simulink model "NLPIDVersion2"  (Simulink 7.3)
settings: Solver=ode5  StartTime=0.0  StopTime=inf  FixedStep=0.1  RelTol=1e-3
undefined symbols (not defined in the file): eta1_0_real, v1_0_real, velocitySatValues1
libraries: dspmtrx3 x16, simulink x14, dspindex x5, marine_gnc x4, simulink_extras x1, dspinverses x1
(part 4 of 4)

== system NLPIDVersion2/Main Subsystems/Guidance/Line-Of-Sight Path-Following/Path/Ellipse path/p_d^s^2 eq ==
  s : Inport
  r_x : Inport  Port=2
  r_y : Inport  Port=3
  k : Inport  Port=4
  Gain : Gain  Gain=-1  ParameterDataType=fixdt(1, 16)  ParameterScaling=2^0  OutDataType=fixdt(1, 16)  OutScaling=2^0
  Gain1 : Gain  Gain=-1  ParameterDataType=fixdt(1, 16)  ParameterScaling=2^0  OutDataType=fixdt(1, 16)  OutScaling=2^0
  Math Function : Math  Operator=square  OutDataType=fixdt(1, 16)  OutScaling=2^0  SaturateOnIntegerOverflow=on
  Mux2 : Mux  Inputs=2
  Product : Product  Inputs=3  OutDataType=fixdt(1, 16)  OutScaling=2^0  RndMeth=Zero
  Product1 : Product  Inputs=3  OutDataType=fixdt(1, 16)  OutScaling=2^0  RndMeth=Zero
  Product2 : Product  OutDataType=fixdt(1, 16)  OutScaling=2^0  RndMeth=Zero
  cos(s) : Trigonometry  Operator=cos
  sin(s) : Trigonometry
  p_d^s^2 : Outport
  wires:
  Math Function/1 -> Product/3, Product1/3
  Product2/1 -> sin(s)/1, cos(s)/1
  s/1 -> Product2/1
  k/1 -> Math Function/1, Product2/2
  r_x/1 -> Product/1
  r_y/1 -> Product1/1
  Mux2/1 -> p_d^s^2/1
  sin(s)/1 -> Product1/2
  cos(s)/1 -> Product/2
  Gain1/1 -> Mux2/2
  Product1/1 -> Gain1/1
  Gain/1 -> Mux2/1
  Product/1 -> Gain/1

== system NLPIDVersion2/Main Subsystems/Guidance/Line-Of-Sight Path-Following/Path/Ellipse path/p_d^s^3 eq ==
  s : Inport
  r_x : Inport  Port=2
  r_y : Inport  Port=3
  k : Inport  Port=4
  Constant : Constant  Value=3  OutDataType=fixdt(1, 16)  OutScaling=2^0
  Gain : Gain  Gain=-1  ParameterDataType=fixdt(1, 16)  ParameterScaling=2^0  OutDataType=fixdt(1, 16)  OutScaling=2^0
  Math Function : Math  Operator=pow  OutDataType=fixdt(1, 16)  OutScaling=2^0  SaturateOnIntegerOverflow=on
  Mux3 : Mux  Inputs=2
  Product : Product  Inputs=3  OutDataType=fixdt(1, 16)  OutScaling=2^0  RndMeth=Zero
  Product1 : Product  Inputs=3  OutDataType=fixdt(1, 16)  OutScaling=2^0  RndMeth=Zero
  Product2 : Product  OutDataType=fixdt(1, 16)  OutScaling=2^0  RndMeth=Zero
  cos(s)3 : Trigonometry  Operator=cos
  sin(s)3 : Trigonometry
  p_d^s^3 : Outport
  wires:
  Math Function/1 -> Product/3, Product1/3
  Constant/1 -> Math Function/2
  Product2/1 -> cos(s)3/1, sin(s)3/1
  s/1 -> Product2/1
  k/1 -> Math Function/1, Product2/2
  r_y/1 -> Product1/1
  r_x/1 -> Product/1
  sin(s)3/1 -> Product/2
  cos(s)3/1 -> Product1/2
  Product/1 -> Mux3/1
  Mux3/1 -> p_d^s^3/1
  Gain/1 -> Mux3/2
  Product1/1 -> Gain/1

== system NLPIDVersion2/Main Subsystems/Guidance/Line-Of-Sight Path-Following/Path/Ellipse path/|p_d^s| eq ==
  p_d^s : Inport
  Product : Product  Multiplication=Matrix(*)  OutDataType=fixdt(1, 16)  OutScaling=2^0  RndMeth=Zero
  p_d^s^T : dspmtrx3/Transpose  SystemSampleTime=-1  Hermitian=off  overflowFlag=off
  sqrt : Math  Operator=sqrt  OutDataType=fixdt(1, 16)  OutScaling=2^0  SaturateOnIntegerOverflow=on
  |p_d^s| : Outport
  wires:
  p_d^s^T/1 -> Product/1
  Product/1 -> sqrt/1
  sqrt/1 -> |p_d^s|/1
  p_d^s/1 -> p_d^s^T/1, Product/2

== system NLPIDVersion2/Main Subsystems/Guidance/Line-Of-Sight Path-Following/Path/Path Switch workaround + limiter/Limiter ==
  p_d : Inport  OutDataType=sfix(16)  OutScaling=2^0
  Demux : Demux  Outputs=2
  Mux1 : Mux  Inputs=2
  Saturation x : simulink/Discontinuities/Saturation Dynamic  SystemSampleTime=-1  OutMin=[]  OutMax=[]  OutDataTypeStr=Inherit: Same as second input  OutDataType=fixdt(1, 16)  OutScaling=2^-10  DoSatur=off
  Saturation y : simulink/Discontinuities/Saturation Dynamic  SystemSampleTime=-1  OutMin=[]  OutMax=[]  OutDataTypeStr=Inherit: Same as second input  OutDataType=fixdt(1, 16)  OutScaling=2^-10  DoSatur=off
  sat_p_d : Outport  PortDimensions=2  OutDataType=sfix(16)  OutScaling=2^0
  wires:
  Saturation y/1 -> Mux1/2
  Saturation x/1 -> Mux1/1
  Demux/2 -> Saturation y/2
  Demux/1 -> Saturation x/2
  p_d/1 -> Demux/1
  Mux1/1 -> sat_p_d/1
  [xdmax] -> Saturation x/1
  [xdmin] -> Saturation x/3
  [ydmax] -> Saturation y/1
  [ydmin] -> Saturation y/3

== system NLPIDVersion2/Main Subsystems/Guidance/Line-Of-Sight Path-Following/Path/Path Switch workaround + limiter/p_d selcetor ==
  note: Path Selector == 1: Linear path
      | Path Selector == 0: Ellipse path
  Path Selector : Inport  OutDataType=fixdt(1, 16)  OutScaling=2^0
  Add : Sum  OutDataType=fixdt(1, 16)  OutScaling=2^-10
  Constant : Constant  OutDataType=fixdt(1, 16)  OutScaling=2^0
  Product : Product  OutDataType=fixdt(1, 16)  OutScaling=2^0  RndMeth=Zero
  Product1 : Product  OutDataType=fixdt(1, 16)  OutScaling=2^0  RndMeth=Zero
  Subract : Sum  Inputs=+-  OutDataType=fixdt(1, 16)  OutScaling=2^-10
  p_d : Outport
  wires:
  Add/1 -> p_d/1
  Path Selector/1 -> Product/2, Subract/2  "chosen path"
  Constant/1 -> Subract/1
  Product/1 -> Add/1
  Subract/1 -> Product1/2
  Product1/1 -> Add/2
  [pdLinear] -> Product/1
  [pdEllipse] -> Product1/1

== system NLPIDVersion2/Main Subsystems/Guidance/Line-Of-Sight Path-Following/Path/Path Switch workaround + limiter/p_d^s selcetor ==
  note: Path Selector == 1: Linear path
      | Path Selector == 0: Ellipse path
  Path Selector : Inport  OutDataType=fixdt(1, 16)  OutScaling=2^0
  Add : Sum  OutDataType=fixdt(1, 16)  OutScaling=2^-10
  Constant : Constant  OutDataType=fixdt(1, 16)  OutScaling=2^0
  Product : Product  OutDataType=fixdt(1, 16)  OutScaling=2^0  RndMeth=Zero
  Product1 : Product  OutDataType=fixdt(1, 16)  OutScaling=2^0  RndMeth=Zero
  Subract : Sum  Inputs=+-  OutDataType=fixdt(1, 16)  OutScaling=2^-10
  p_d^s : Outport
  wires:
  [pd_sEllipse] -> Product1/1
  [pd_sLinear] -> Product/1
  Product1/1 -> Add/2
  Subract/1 -> Product1/2
  Product/1 -> Add/1
  Constant/1 -> Subract/1
  Path Selector/1 -> Subract/2, Product/2  "chosen path"
  Add/1 -> p_d^s/1

== system NLPIDVersion2/Main Subsystems/Guidance/Line-Of-Sight Path-Following/Path/Path Switch workaround + limiter/p_d^s^2 selcetor ==
  note: Path Selector == 1: Linear path
      | Path Selector == 0: Ellipse path
  Path Selector : Inport  OutDataType=fixdt(1, 16)  OutScaling=2^0
  Add : Sum  OutDataType=fixdt(1, 16)  OutScaling=2^-10
  Constant : Constant  OutDataType=fixdt(1, 16)  OutScaling=2^0
  Product : Product  OutDataType=fixdt(1, 16)  OutScaling=2^0  RndMeth=Zero
  Product1 : Product  OutDataType=fixdt(1, 16)  OutScaling=2^0  RndMeth=Zero
  Subract : Sum  Inputs=+-  OutDataType=fixdt(1, 16)  OutScaling=2^-10
  p_d^s^2 : Outport
  wires:
  Add/1 -> p_d^s^2/1
  Path Selector/1 -> Product/2, Subract/2  "chosen path"
  Constant/1 -> Subract/1
  Product/1 -> Add/1
  Subract/1 -> Product1/2
  Product1/1 -> Add/2
  [pd_s_2Linear] -> Product/1
  [pd_s_2Ellipse] -> Product1/1

== system NLPIDVersion2/Main Subsystems/Guidance/Line-Of-Sight Path-Following/Path/Path Switch workaround + limiter/p_d^s^3 selcetor ==
  note: Path Selector == 1: Linear path
      | Path Selector == 0: Ellipse path
  Path Selector : Inport  OutDataType=fixdt(1, 16)  OutScaling=2^0
  Add : Sum  OutDataType=fixdt(1, 16)  OutScaling=2^-10
  Constant : Constant  OutDataType=fixdt(1, 16)  OutScaling=2^0
  Product : Product  OutDataType=fixdt(1, 16)  OutScaling=2^0  RndMeth=Zero
  Product1 : Product  OutDataType=fixdt(1, 16)  OutScaling=2^0  RndMeth=Zero
  Subract : Sum  Inputs=+-  OutDataType=fixdt(1, 16)  OutScaling=2^-10
  p_d^s^3 : Outport
  wires:
  [pd_s_3Ellipse] -> Product1/1
  [pd_s_3Linear] -> Product/1
  Product1/1 -> Add/2
  Subract/1 -> Product1/2
  Product/1 -> Add/1
  Constant/1 -> Subract/1
  Path Selector/1 -> Subract/2, Product/2  "chosen path"
  Add/1 -> p_d^s^3/1

== system NLPIDVersion2/Main Subsystems/Guidance/Line-Of-Sight Path-Following/Path/Path Switch workaround + limiter/p_d^s^3 selcetor1 ==
  note: Path Selector == 1: Linear path
      | Path Selector == 0: Ellipse path
  Path Selector : Inport  OutDataType=fixdt(1, 16)  OutScaling=2^0
  Add : Sum  OutDataType=fixdt(1, 16)  OutScaling=2^-10
  Constant : Constant  OutDataType=fixdt(1, 16)  OutScaling=2^0
  Product : Product  OutDataType=fixdt(1, 16)  OutScaling=2^0  RndMeth=Zero
  Product1 : Product  OutDataType=fixdt(1, 16)  OutScaling=2^0  RndMeth=Zero
  Subract : Sum  Inputs=+-  OutDataType=fixdt(1, 16)  OutScaling=2^-10
  |p_d^s| : Outport
  wires:
  Add/1 -> |p_d^s|/1
  Path Selector/1 -> Product/2, Subract/2  "chosen path"
  Constant/1 -> Subract/1
  Product/1 -> Add/1
  Subract/1 -> Product1/2
  Product1/1 -> Add/2
  [pd_sabsLinear] -> Product/1
  [pd_sabsEllipse] -> Product1/1

== system NLPIDVersion2/Main Subsystems/Guidance/Line-Of-Sight Path-Following/Path/Straight path/p_d eq ==
  s : Inport
  x_1 : Inport  Port=2
  y_1 : Inport  Port=3
  x_2 : Inport  Port=4
  y_2 : Inport  Port=5
  (x_2 - x_1) * s : Product  OutDataType=fixdt(1, 16)  OutScaling=2^0  RndMeth=Zero
  (x_2 - x_1) * s + x_1 : Sum  OutDataType=fixdt(1, 16)  OutScaling=2^-10
  (y_2 - y_1) * s : Product  OutDataType=fixdt(1, 16)  OutScaling=2^0  RndMeth=Zero
  (y_2 - y_1) * s + y_1 : Sum  OutDataType=fixdt(1, 16)  OutScaling=2^-10
  Mux1 : Mux  Inputs=2
  x_2 - x_1 : Sum  Inputs=+-  OutDataType=fixdt(1, 16)  OutScaling=2^-10
  y_2 - y_1 : Sum  Inputs=+-  OutDataType=fixdt(1, 16)  OutScaling=2^-10
  p_d : Outport
  wires:
  Mux1/1 -> p_d/1
  y_1/1 -> (y_2 - y_1) * s + y_1/2, y_2 - y_1/2
  y_2/1 -> y_2 - y_1/1
  x_1/1 -> (x_2 - x_1) * s + x_1/2, x_2 - x_1/2
  x_2/1 -> x_2 - x_1/1
  s/1 -> (y_2 - y_1) * s/2, (x_2 - x_1) * s/2
  y_2 - y_1/1 -> (y_2 - y_1) * s/1
  x_2 - x_1/1 -> (x_2 - x_1) * s/1
  (y_2 - y_1) * s/1 -> (y_2 - y_1) * s + y_1/1
  (x_2 - x_1) * s/1 -> (x_2 - x_1) * s + x_1/1
  (y_2 - y_1) * s + y_1/1 -> Mux1/2
  (x_2 - x_1) * s + x_1/1 -> Mux1/1

== system NLPIDVersion2/Main Subsystems/Guidance/Line-Of-Sight Path-Following/Path/Straight path/p_d^s eq ==
  x_1 : Inport
  y_1 : Inport  Port=2
  x_2 : Inport  Port=3
  y_2 : Inport  Port=4
  Mux1 : Mux  Inputs=2
  x_2 - x_1 : Sum  Inputs=+-  OutDataType=fixdt(1, 16)  OutScaling=2^-10
  y_2 - y_1 : Sum  Inputs=+-  OutDataType=fixdt(1, 16)  OutScaling=2^-10
  p_d^s : Outport
  wires:
  y_1/1 -> y_2 - y_1/2
  y_2/1 -> y_2 - y_1/1
  x_1/1 -> x_2 - x_1/2
  x_2/1 -> x_2 - x_1/1
  y_2 - y_1/1 -> Mux1/2
  x_2 - x_1/1 -> Mux1/1
  Mux1/1 -> p_d^s/1

== system NLPIDVersion2/Main Subsystems/Guidance/Line-Of-Sight Path-Following/Path/Straight path/|p_d^s| eq ==
  p_d^s : Inport
  Product : Product  Multiplication=Matrix(*)  OutDataType=fixdt(1, 16)  OutScaling=2^0  RndMeth=Zero
  p_d^s^T : dspmtrx3/Transpose  SystemSampleTime=-1  Hermitian=off  overflowFlag=off
  sqrt : Math  Operator=sqrt  OutDataType=fixdt(1, 16)  OutScaling=2^0  SaturateOnIntegerOverflow=on
  |p_d^s| : Outport
  wires:
  p_d^s/1 -> Product/2, p_d^s^T/1
  sqrt/1 -> |p_d^s|/1
  Product/1 -> sqrt/1
  p_d^s^T/1 -> Product/1

== system NLPIDVersion2/Main Subsystems/Guidance/Line-Of-Sight Path-Following/Line-Of-Sight/LOS heading/psi_los eq/rad to [-pi pi] ==
  rad : Inport  OutDataType=sfix(16)  OutScaling=2^0
  Constant : Constant  Value=2*pi  OutDataType=sfix(16)  OutScaling=2^0
  Gain : Gain  Gain=pi  ParameterDataType=sfix(16)  ParameterScaling=2^0  OutDataType=sfix(16)  OutScaling=2^0  SaturateOnIntegerOverflow=on  OutDataTypeStr=Inherit: Same as input  ParamDataTypeStr=Inherit: Same as input
  Math Function : Math  Operator=rem  OutDataType=sfix(16)  OutScaling=2^0  SaturateOnIntegerOverflow=on
  Saturation : Saturate  UpperLimit=1e10  LowerLimit=-1e10
  Sign : Signum
  Sum : Sum  Inputs=|+-  OutDataType=sfix(16)  OutScaling=2^0  SaturateOnIntegerOverflow=on
  Sum1 : Sum  Inputs=|++  OutDataType=sfix(16)  OutScaling=2^0  SaturateOnIntegerOverflow=on
  "[-pi pi]" : Outport  OutDataType=sfix(16)  OutScaling=2^0
  wires:
  Sum/1 -> "[-pi pi]"/1
  Math Function/1 -> Sum/1
  Constant/1 -> Math Function/2
  Sum1/1 -> Math Function/1
  Gain/1 -> Sum1/2, Sum/2
  Sign/1 -> Gain/1
  rad/1 -> Saturation/1
  Saturation/1 -> Sign/1, Sum1/1

== system NLPIDVersion2/Main Subsystems/Guidance/Line-Of-Sight Path-Following/Line-Of-Sight/LOS heading/psi_los eq/rad to [-pi pi]1 ==
  rad : Inport  OutDataType=sfix(16)  OutScaling=2^0
  Constant : Constant  Value=2*pi  OutDataType=sfix(16)  OutScaling=2^0
  Gain : Gain  Gain=pi  ParameterDataType=sfix(16)  ParameterScaling=2^0  OutDataType=sfix(16)  OutScaling=2^0  SaturateOnIntegerOverflow=on  OutDataTypeStr=Inherit: Same as input  ParamDataTypeStr=Inherit: Same as input
  Math Function : Math  Operator=rem  OutDataType=sfix(16)  OutScaling=2^0  SaturateOnIntegerOverflow=on
  Saturation : Saturate  UpperLimit=1e10  LowerLimit=-1e10
  Sign : Signum
  Sum : Sum  Inputs=|+-  OutDataType=sfix(16)  OutScaling=2^0  SaturateOnIntegerOverflow=on
  Sum1 : Sum  Inputs=|++  OutDataType=sfix(16)  OutScaling=2^0  SaturateOnIntegerOverflow=on
  "[-pi pi]" : Outport  OutDataType=sfix(16)  OutScaling=2^0
  wires:
  Saturation/1 -> Sum1/1, Sign/1
  rad/1 -> Saturation/1
  Sign/1 -> Gain/1
  Gain/1 -> Sum/2, Sum1/2
  Sum1/1 -> Math Function/1
  Constant/1 -> Math Function/2
  Math Function/1 -> Sum/1
  Sum/1 -> "[-pi pi]"/1

== system NLPIDVersion2/Main Subsystems/Guidance/Line-Of-Sight Path-Following/Line-Of-Sight/LOS heading/psi_los eq/rad to [-pi pi]2 ==
  rad : Inport  OutDataType=sfix(16)  OutScaling=2^0
  Constant : Constant  Value=2*pi  OutDataType=sfix(16)  OutScaling=2^0
  Gain : Gain  Gain=pi  ParameterDataType=sfix(16)  ParameterScaling=2^0  OutDataType=sfix(16)  OutScaling=2^0  SaturateOnIntegerOverflow=on  OutDataTypeStr=Inherit: Same as input  ParamDataTypeStr=Inherit: Same as input
  Math Function : Math  Operator=rem  OutDataType=sfix(16)  OutScaling=2^0  SaturateOnIntegerOverflow=on
  Saturation : Saturate  UpperLimit=1e10  LowerLimit=-1e10
  Sign : Signum
  Sum : Sum  Inputs=|+-  OutDataType=sfix(16)  OutScaling=2^0  SaturateOnIntegerOverflow=on
  Sum1 : Sum  Inputs=|++  OutDataType=sfix(16)  OutScaling=2^0  SaturateOnIntegerOverflow=on
  "[-pi pi]" : Outport  OutDataType=sfix(16)  OutScaling=2^0
  wires:
  Sum/1 -> "[-pi pi]"/1
  Math Function/1 -> Sum/1
  Constant/1 -> Math Function/2
  Sum1/1 -> Math Function/1
  Gain/1 -> Sum1/2, Sum/2
  Sign/1 -> Gain/1
  rad/1 -> Saturation/1
  Saturation/1 -> Sign/1, Sum1/1
